simulink model "lab4_2"  (R2021b)
settings: Solver=ode4  StartTime=0.0  StopTime=100.0  FixedStep=0.04  RelTol=1e-3
settings Model: Creator=JaSzw  LastModifiedBy=JaSzw

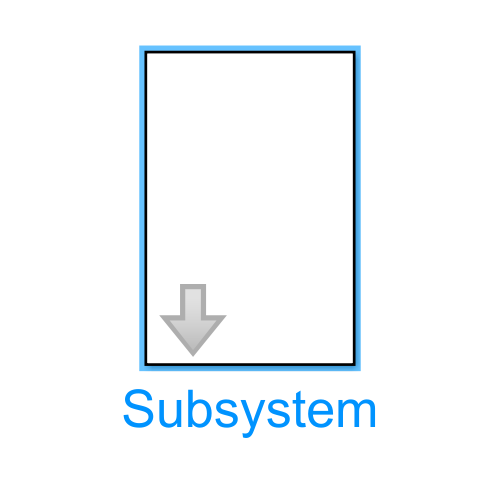
[thumbnail: Simulink's stored preview of the top-level diagram]
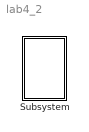
== system lab4_2 ==
  Subsystem : Subsystem  mask{m=10, l=3, g=10, k=1, ph0=90, ph1=100}
      mask prompts: m "masa"; l "długość"; g "grawitacja"; k "tłumenie"; ph0 "kąt pocz."; ph1 "prędkość"

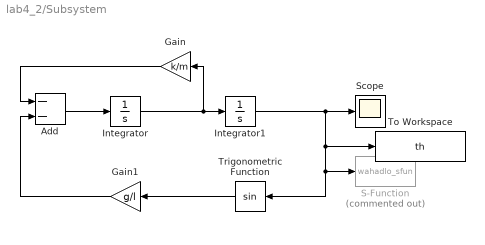
== system lab4_2/Subsystem ==
  Add : Sum  Inputs=--
  Gain : Gain  Gain=k/m
  Gain1 : Gain  Gain=g/l
  Integrator : Integrator  InitialCondition=ph1*pi/180
  Integrator1 : Integrator  InitialCondition=ph0*pi/180
  S-Function : S-Function  Commented=on  FunctionName=wahadlo_sfun  Parameters=l,m,ph0  SFunctionDeploymentMode=off  EnableBusSupport=off
  Scope : Scope
  To Workspace : ToWorkspace  VariableName=th  SampleTime=-1
  Trigonometric Function : Trigonometry
  wires:
  Add/1 -> Integrator/1
  Integrator1/1 -> Scope/1, To Workspace/1, S-Function/1, Trigonometric Function/1
  Trigonometric Function/1 -> Gain1/1
  Gain1/1 -> Add/2
  Integrator/1 -> Gain/1, Integrator1/1
  Gain/1 -> Add/1
